simulink model "Ex4_11"  (Simulink 6.0)
settings: Solver=VariableStepDiscrete  StartTime=0.0  StopTime=Tstop  RelTol=1e-3
values from neighbouring files (symbols this model uses):
  Ampl = 10^(Amp_dB/20)*Vfs/2    (= 1)    [Ex4_11_launch.m]
  finrad = Fin*2*pi    (= 11198059.7516)    [Ex4_11_launch.m]
  gain = 1    [Ex4_11_launch.m]
  GAIN1 = 2.0    (= 2)    [Ex4_11_launch.m]
  gain1 = 1    [Ex4_11_launch.m]
  GAIN2 = 2.0    (= 2)    [Ex4_11_launch.m]
  gain2 = 1    [Ex4_11_launch.m]
  GAIN3 = 2.0    (= 2)    [Ex4_11_launch.m]
  gainH = 1    [Ex4_11_launch.m]
  sr = 25000e8    (= 2500000000000)    [Ex4_11_launch.m]
  sr1 = 10000e8    (= 1000000000000)    [Ex4_11_launch.m]
  sr2 = 20000e8    (= 2000000000000)    [Ex4_11_launch.m]
  srH = 250e6    (= 250000000)    [Ex4_11_launch.m]
  tau = 1/(2*pi*beta*f_T)    (= 5.30516476973e-11)    [Ex4_11_launch.m]
  tau1 = 1/(2*pi*beta1*f_T1)    (= 5.30516476973e-11)    [Ex4_11_launch.m]
  tau2 = 1/(2*pi*beta2*f_T2)    (= 5.30516476973e-11)    [Ex4_11_launch.m]
  tauH = 1/(2*pi*betaH*f_TH)    (= 2.65258238486e-10)    [Ex4_11_launch.m]
  Tmax = Ts/2    (= 5e-09)    [Ex4_11_launch.m]
  Ts = 1e-8    (= 1e-08)    [Ex4_11_launch.m]
  V_DAC_H1 = 0.5    [Ex4_11_launch.m]
  V_DAC_H2 = 0.5    [Ex4_11_launch.m]
  V_DAC_H3 = 0.5    [Ex4_11_launch.m]
  V_DAC_L1 = -0.5    [Ex4_11_launch.m]
  V_DAC_L2 = -0.5    [Ex4_11_launch.m]
  V_DAC_L3 = -0.5    [Ex4_11_launch.m]
  VthH1 = 0.25+eps    [Ex4_11_launch.m]
  VthH2 = 0.25+eps    [Ex4_11_launch.m]
  VthH3 = 0.25+eps    [Ex4_11_launch.m]
  VthL1 = -0.25+eps    [Ex4_11_launch.m]
  VthL2 = -0.25+eps    [Ex4_11_launch.m]
  VthL3 = -0.25+eps    [Ex4_11_launch.m]
undefined symbols (not defined in the file or in its folder): RealBuffer
settings Model: Creator=francomaloberti  LastModifiedBy=Cri  ExtModeAutoUpdateStatusClock=off
settings DataIOCC: SignalLoggingName=sigsOut
settings OptimizationCC: InlineInvariantSignals=off
settings DebuggingCC: SolverPrmCheckMsg=none
settings HardwareCC: TargetUnknown=on

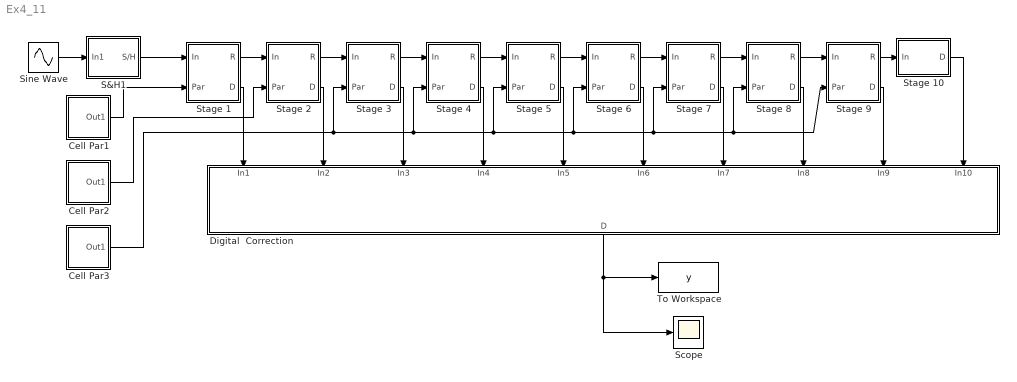
== system Ex4_11 ==
  Cell Par1 : Subsystem
  Cell Par2 : Subsystem
  Cell Par3 : Subsystem
  Digital  Correction : Subsystem  Orientation=down
  S&H1 : Subsystem
  Scope : Scope
  Sine Wave : Sin  Amplitude=Ampl  Frequency=finrad  SampleTime=0
  Stage 1 : Subsystem
  Stage 10 : Subsystem
  Stage 2 : Subsystem
  Stage 3 : Subsystem
  Stage 4 : Subsystem
  Stage 5 : Subsystem
  Stage 6 : Subsystem
  Stage 7 : Subsystem
  Stage 8 : Subsystem
  Stage 9 : Subsystem
  To Workspace : ToWorkspace  VariableName=y  SampleTime=-1  SaveFormat=Array
  wires:
  S&H1/1(S/H) -> Stage 1/1(In)
  Stage 1/1(R) -> Stage 2/1(In)
  Stage 2/1(R) -> Stage 3/1(In)
  Stage 3/1(R) -> Stage 4/1(In)
  Stage 4/1(R) -> Stage 5/1(In)
  Stage 5/1(R) -> Stage 6/1(In)
  Stage 6/1(R) -> Stage 7/1(In)
  Stage 7/1(R) -> Stage 8/1(In)
  Stage 8/1(R) -> Stage 9/1(In)
  Stage 9/1(R) -> Stage 10/1(In)
  Stage 9/2(D) -> Digital  Correction/9(In9)
  Stage 8/2(D) -> Digital  Correction/8(In8)
  Stage 7/2(D) -> Digital  Correction/7(In7)
  Stage 6/2(D) -> Digital  Correction/6(In6)
  Stage 4/2(D) -> Digital  Correction/4(In4)
  Stage 3/2(D) -> Digital  Correction/3(In3)
  Stage 2/2(D) -> Digital  Correction/2(In2)
  Stage 1/2(D) -> Digital  Correction/1(In1)
  Stage 5/2(D) -> Digital  Correction/5(In5)
  Cell Par1/1(Out1) -> Stage 1/2(Par)
  Cell Par2/1(Out1) -> Stage 2/2(Par)
  Cell Par3/1(Out1) -> Stage 3/2(Par), Stage 4/2(Par), Stage 5/2(Par), Stage 6/2(Par), Stage 8/2(Par), Stage 9/2(Par), Stage 7/2(Par)
  Stage 10/1(D) -> Digital  Correction/10(In10)
  Sine Wave/1 -> S&H1/1(In1)
  Digital  Correction/1(D) -> To Workspace/1, Scope/1

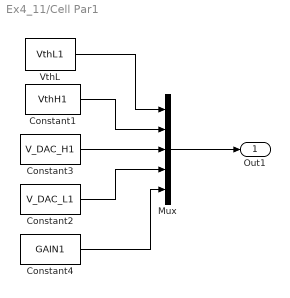
== system Ex4_11/Cell Par1 ==
  Constant1 : Constant  Value=VthH1
  Constant2 : Constant  Value=V_DAC_L1
  Constant3 : Constant  Value=V_DAC_H1
  Constant4 : Constant  Value=GAIN1
  Mux : Mux  Inputs=5
  VthL : Constant  Value=VthL1
  Out1 : Outport
  wires:
  Mux/1 -> Out1/1
  VthL/1 -> Mux/1
  Constant1/1 -> Mux/2
  Constant4/1 -> Mux/5
  Constant3/1 -> Mux/3
  Constant2/1 -> Mux/4

== system Ex4_11/Cell Par2 ==
  Constant1 : Constant  Value=VthH2
  Constant2 : Constant  Value=V_DAC_L2
  Constant3 : Constant  Value=V_DAC_H2
  Constant4 : Constant  Value=GAIN2
  Mux : Mux  Inputs=5
  VthL : Constant  Value=VthL2
  Out1 : Outport
  wires:
  Constant2/1 -> Mux/4
  Constant3/1 -> Mux/3
  Constant4/1 -> Mux/5
  Constant1/1 -> Mux/2
  VthL/1 -> Mux/1
  Mux/1 -> Out1/1

== system Ex4_11/Cell Par3 ==
  Constant1 : Constant  Value=VthH3
  Constant2 : Constant  Value=V_DAC_L3
  Constant3 : Constant  Value=V_DAC_H3
  Constant4 : Constant  Value=GAIN3
  Mux : Mux  Inputs=5
  VthL : Constant  Value=VthL3
  Out1 : Outport
  wires:
  Mux/1 -> Out1/1
  VthL/1 -> Mux/1
  Constant1/1 -> Mux/2
  Constant4/1 -> Mux/5
  Constant3/1 -> Mux/3
  Constant2/1 -> Mux/4

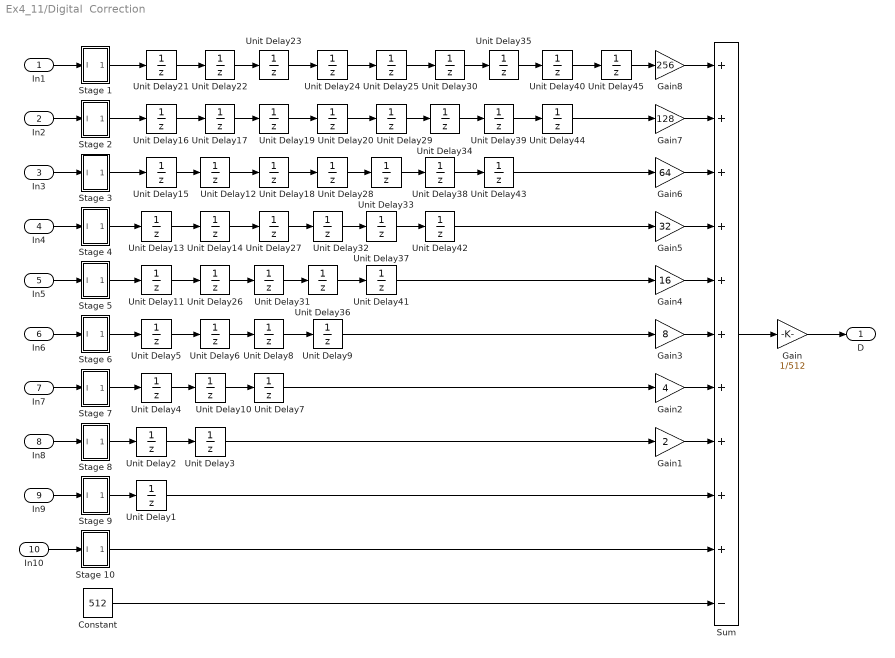
== system Ex4_11/Digital  Correction ==
  In1 : Inport  Port=1  LatchInput=off
  In2 : Inport  Port=2  LatchInput=off
  In3 : Inport  Port=3  LatchInput=off
  In4 : Inport  Port=4  LatchInput=off
  In5 : Inport  Port=5  LatchInput=off
  In6 : Inport  Port=6  LatchInput=off
  In7 : Inport  Port=7  LatchInput=off
  In8 : Inport  Port=8  LatchInput=off
  In9 : Inport  Port=9  LatchInput=off
  In10 : Inport  Port=10  LatchInput=off
  Constant : Constant  Value=512
  Gain : Gain  Gain=1/512
  Gain1 : Gain  Gain=2
  Gain2 : Gain  Gain=4
  Gain3 : Gain  Gain=8
  Gain4 : Gain  Gain=16
  Gain5 : Gain  Gain=32
  Gain6 : Gain  Gain=64
  Gain7 : Gain  Gain=128
  Gain8 : Gain  Gain=256
  Stage 1 : Subsystem
  Stage 10 : Subsystem
  Stage 2 : Subsystem
  Stage 3 : Subsystem
  Stage 4 : Subsystem
  Stage 5 : Subsystem
  Stage 6 : Subsystem
  Stage 7 : Subsystem
  Stage 8 : Subsystem
  Stage 9 : Subsystem
  Sum : Sum  Inputs=++++++++++-
  Unit Delay{1..45} (45 alike) : UnitDelay  SampleTime=Ts
  D : Outport
  wires:
  Gain8/1 -> Sum/1
  Gain7/1 -> Sum/2
  Gain6/1 -> Sum/3
  Gain5/1 -> Sum/4
  Gain4/1 -> Sum/5
  Gain3/1 -> Sum/6
  Gain2/1 -> Sum/7
  Gain1/1 -> Sum/8
  Constant/1 -> Sum/11
  Stage 10/1(D) -> Sum/10
  Unit Delay1/1 -> Sum/9
  Unit Delay3/1 -> Gain1/1
  Unit Delay7/1 -> Gain2/1
  Unit Delay9/1 -> Gain3/1
  Unit Delay41/1 -> Gain4/1
  Unit Delay42/1 -> Gain5/1
  Unit Delay43/1 -> Gain6/1
  Unit Delay44/1 -> Gain7/1
  Unit Delay45/1 -> Gain8/1
  Unit Delay40/1 -> Unit Delay45/1
  Unit Delay35/1 -> Unit Delay40/1
  Unit Delay30/1 -> Unit Delay35/1
  Unit Delay25/1 -> Unit Delay30/1
  Unit Delay39/1 -> Unit Delay44/1
  Unit Delay34/1 -> Unit Delay39/1
  Unit Delay29/1 -> Unit Delay34/1
  Unit Delay20/1 -> Unit Delay29/1
  Unit Delay38/1 -> Unit Delay43/1
  Unit Delay33/1 -> Unit Delay38/1
  Unit Delay28/1 -> Unit Delay33/1
  Unit Delay18/1 -> Unit Delay28/1
  Unit Delay37/1 -> Unit Delay42/1
  Unit Delay32/1 -> Unit Delay37/1
  Unit Delay27/1 -> Unit Delay32/1
  Unit Delay14/1 -> Unit Delay27/1
  Unit Delay36/1 -> Unit Delay41/1
  Unit Delay31/1 -> Unit Delay36/1
  Unit Delay26/1 -> Unit Delay31/1
  Unit Delay11/1 -> Unit Delay26/1
  Unit Delay24/1 -> Unit Delay25/1
  Stage 1/1(D) -> Unit Delay21/1
  Unit Delay22/1 -> Unit Delay23/1
  Unit Delay23/1 -> Unit Delay24/1
  Unit Delay21/1 -> Unit Delay22/1
  Stage 2/1(D) -> Unit Delay16/1
  Stage 3/1(D) -> Unit Delay15/1
  Stage 4/1(D) -> Unit Delay13/1
  Stage 5/1(D) -> Unit Delay11/1
  Unit Delay17/1 -> Unit Delay19/1
  Unit Delay12/1 -> Unit Delay18/1
  Unit Delay15/1 -> Unit Delay12/1
  Unit Delay19/1 -> Unit Delay20/1
  Unit Delay16/1 -> Unit Delay17/1
  Unit Delay13/1 -> Unit Delay14/1
  Unit Delay6/1 -> Unit Delay8/1
  Stage 6/1(D) -> Unit Delay5/1
  Unit Delay10/1 -> Unit Delay7/1
  Unit Delay4/1 -> Unit Delay10/1
  Stage 7/1(D) -> Unit Delay4/1
  Unit Delay8/1 -> Unit Delay9/1
  Unit Delay5/1 -> Unit Delay6/1
  Stage 9/1(D) -> Unit Delay1/1
  Unit Delay2/1 -> Unit Delay3/1
  Stage 8/1(D) -> Unit Delay2/1
  In9/1 -> Stage 9/1(I)
  In8/1 -> Stage 8/1(I)
  In7/1 -> Stage 7/1(I)
  In6/1 -> Stage 6/1(I)
  In5/1 -> Stage 5/1(I)
  In4/1 -> Stage 4/1(I)
  In3/1 -> Stage 3/1(I)
  In2/1 -> Stage 2/1(I)
  In1/1 -> Stage 1/1(I)
  In10/1 -> Stage 10/1(I)
  Gain/1 -> D/1
  Sum/1 -> Gain/1

== system Ex4_11/S&H1 ==
  In1 : Inport  Port=1  LatchInput=off
  Constant : Constant  Value=1/1024-eps
  MATLAB Fcn : MATLABFcn  MATLABFcn=RealBuffer(u,srH,tauH,gainH,Tmax)
  Sum1 : Sum  Inputs=|++  SaturateOnIntegerOverflow=on
  Unit Delay1 : UnitDelay  SampleTime=Ts
  S/H : Outport
  wires:
  Constant/1 -> Sum1/2
  Unit Delay1/1 -> Sum1/1
  Sum1/1 -> MATLAB Fcn/1
  In1/1 -> Unit Delay1/1
  MATLAB Fcn/1 -> S/H/1

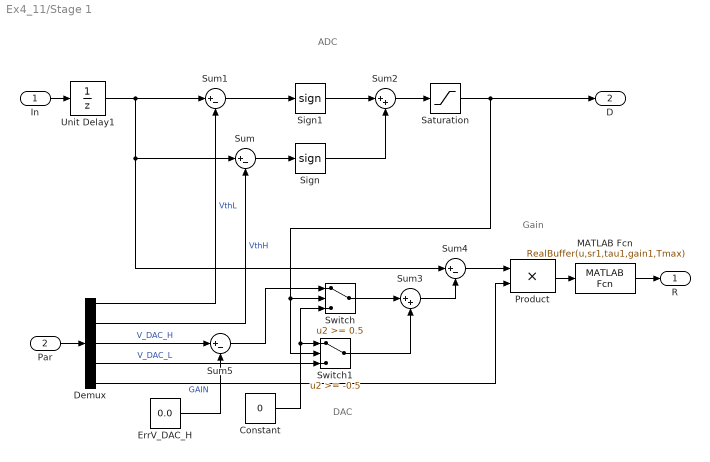
== system Ex4_11/Stage 1 ==
  note: ADC
  note: DAC
  note: Gain
  In : Inport  Port=1  LatchInput=off
  Par : Inport  Port=2  LatchInput=off
  Constant : Constant  Value=0
  Demux : Demux  Outputs=5
  ErrV_DAC_H : Constant  Value=0.0
  MATLAB Fcn : MATLABFcn  MATLABFcn=RealBuffer(u,sr1,tau1,gain1,Tmax)
  Product : Product  SaturateOnIntegerOverflow=on
  Saturation : Saturate  UpperLimit=1  LowerLimit=-1
  Sign : Signum
  Sign1 : Signum
  Sum{,1,4..5} (4 alike) : Sum  Inputs=|+-  SaturateOnIntegerOverflow=on
  Sum2 : Sum  Inputs=|++  SaturateOnIntegerOverflow=on
  Sum3 : Sum  Inputs=|++  SaturateOnIntegerOverflow=on
  Switch : Switch  Threshold=0.5  SaturateOnIntegerOverflow=on
  Switch1 : Switch  Threshold=-0.5  SaturateOnIntegerOverflow=on
  Unit Delay1 : UnitDelay  SampleTime=Ts
  R : Outport
  D : Outport  Port=2
  wires:
  Par/1 -> Demux/1
  Sum/1 -> Sign/1
  Sum1/1 -> Sign1/1
  Demux/1 -> Sum1/2  "VthL"
  Demux/2 -> Sum/2  "VthH"
  In/1 -> Unit Delay1/1
  Sign1/1 -> Sum2/1
  Sign/1 -> Sum2/2
  Sum2/1 -> Saturation/1
  Saturation/1 -> Switch1/2, Switch/2, D/1
  Switch/1 -> Sum3/1
  Switch1/1 -> Sum3/2
  Demux/4 -> Switch1/3  "V_DAC_L"
  Constant/1 -> Switch/3, Switch1/1
  Demux/5 -> Product/2  "GAIN"
  Product/1 -> MATLAB Fcn/1
  Sum3/1 -> Sum4/2
  Sum4/1 -> Product/1
  Demux/3 -> Sum5/1  "V_DAC_H"
  Sum5/1 -> Switch/1
  ErrV_DAC_H/1 -> Sum5/2
  Unit Delay1/1 -> Sum1/1, Sum4/1, Sum/1
  MATLAB Fcn/1 -> R/1

== system Ex4_11/Stage 10 ==
  note: ADC
  In : Inport  Port=1  LatchInput=off
  Sign1 : Signum
  Unit Delay1 : UnitDelay  SampleTime=Ts
  D : Outport
  wires:
  Unit Delay1/1 -> Sign1/1
  Sign1/1 -> D/1
  In/1 -> Unit Delay1/1

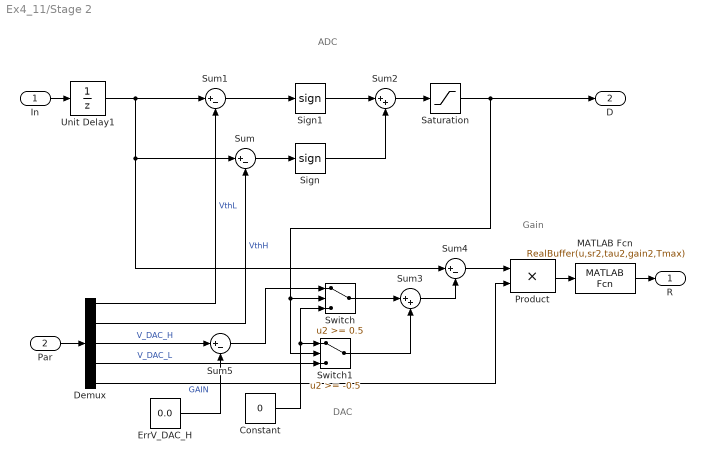
== system Ex4_11/Stage 2 ==
  note: Gain
  note: DAC
  note: ADC
  In : Inport  Port=1  LatchInput=off
  Par : Inport  Port=2  LatchInput=off
  Constant : Constant  Value=0
  Demux : Demux  Outputs=5
  ErrV_DAC_H : Constant  Value=0.0
  MATLAB Fcn : MATLABFcn  MATLABFcn=RealBuffer(u,sr2,tau2,gain2,Tmax)
  Product : Product  SaturateOnIntegerOverflow=on
  Saturation : Saturate  UpperLimit=1  LowerLimit=-1
  Sign : Signum
  Sign1 : Signum
  Sum{,1,4..5} (4 alike) : Sum  Inputs=|+-  SaturateOnIntegerOverflow=on
  Sum2 : Sum  Inputs=|++  SaturateOnIntegerOverflow=on
  Sum3 : Sum  Inputs=|++  SaturateOnIntegerOverflow=on
  Switch : Switch  Threshold=0.5  SaturateOnIntegerOverflow=on
  Switch1 : Switch  Threshold=-0.5  SaturateOnIntegerOverflow=on
  Unit Delay1 : UnitDelay  SampleTime=Ts
  R : Outport
  D : Outport  Port=2
  wires:
  Unit Delay1/1 -> Sum/1, Sum4/1, Sum1/1
  ErrV_DAC_H/1 -> Sum5/2
  Sum5/1 -> Switch/1
  Demux/3 -> Sum5/1  "V_DAC_H"
  Sum4/1 -> Product/1
  Sum3/1 -> Sum4/2
  Product/1 -> MATLAB Fcn/1
  Demux/5 -> Product/2  "GAIN"
  Constant/1 -> Switch1/1, Switch/3
  Demux/4 -> Switch1/3  "V_DAC_L"
  Switch1/1 -> Sum3/2
  Switch/1 -> Sum3/1
  Saturation/1 -> D/1, Switch/2, Switch1/2
  Sum2/1 -> Saturation/1
  Sign/1 -> Sum2/2
  Sign1/1 -> Sum2/1
  In/1 -> Unit Delay1/1
  Demux/2 -> Sum/2  "VthH"
  Demux/1 -> Sum1/2  "VthL"
  Sum1/1 -> Sign1/1
  Sum/1 -> Sign/1
  Par/1 -> Demux/1
  MATLAB Fcn/1 -> R/1

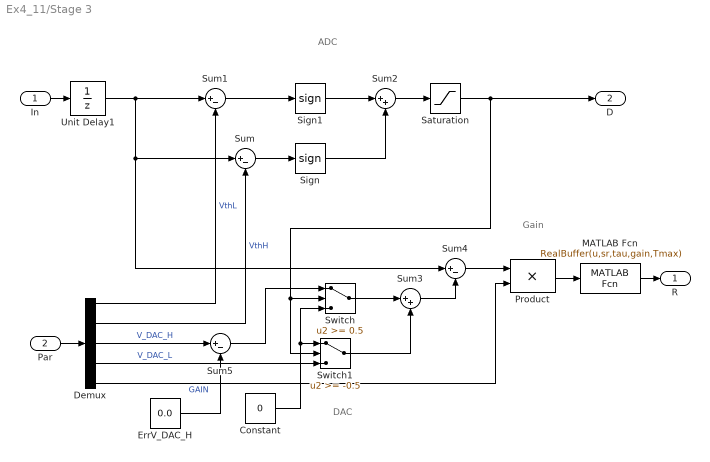
== system Ex4_11/Stage 3 ==
  note: ADC
  note: DAC
  note: Gain
  In : Inport  Port=1  LatchInput=off
  Par : Inport  Port=2  LatchInput=off
  Constant : Constant  Value=0
  Demux : Demux  Outputs=5
  ErrV_DAC_H : Constant  Value=0.0
  MATLAB Fcn : MATLABFcn  MATLABFcn=RealBuffer(u,sr,tau,gain,Tmax)
  Product : Product  SaturateOnIntegerOverflow=on
  Saturation : Saturate  UpperLimit=1  LowerLimit=-1
  Sign : Signum
  Sign1 : Signum
  Sum{,1,4..5} (4 alike) : Sum  Inputs=|+-  SaturateOnIntegerOverflow=on
  Sum2 : Sum  Inputs=|++  SaturateOnIntegerOverflow=on
  Sum3 : Sum  Inputs=|++  SaturateOnIntegerOverflow=on
  Switch : Switch  Threshold=0.5  SaturateOnIntegerOverflow=on
  Switch1 : Switch  Threshold=-0.5  SaturateOnIntegerOverflow=on
  Unit Delay1 : UnitDelay  SampleTime=Ts
  R : Outport
  D : Outport  Port=2
  wires:
  Par/1 -> Demux/1
  Sum/1 -> Sign/1
  Sum1/1 -> Sign1/1
  Demux/1 -> Sum1/2  "VthL"
  Demux/2 -> Sum/2  "VthH"
  In/1 -> Unit Delay1/1
  Sign1/1 -> Sum2/1
  Sign/1 -> Sum2/2
  Sum2/1 -> Saturation/1
  Saturation/1 -> Switch1/2, Switch/2, D/1
  Switch/1 -> Sum3/1
  Switch1/1 -> Sum3/2
  Demux/4 -> Switch1/3  "V_DAC_L"
  Constant/1 -> Switch/3, Switch1/1
  Demux/5 -> Product/2  "GAIN"
  Product/1 -> MATLAB Fcn/1
  Sum3/1 -> Sum4/2
  Sum4/1 -> Product/1
  Demux/3 -> Sum5/1  "V_DAC_H"
  Sum5/1 -> Switch/1
  ErrV_DAC_H/1 -> Sum5/2
  Unit Delay1/1 -> Sum1/1, Sum4/1, Sum/1
  MATLAB Fcn/1 -> R/1

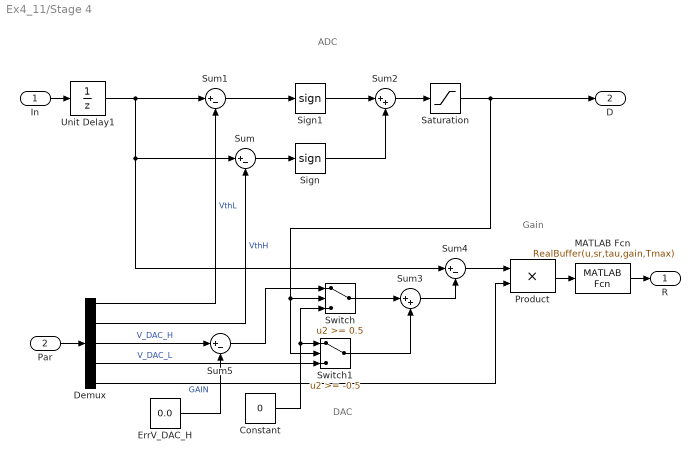
== system Ex4_11/Stage 4 ==
  note: Gain
  note: DAC
  note: ADC
  In : Inport  Port=1  LatchInput=off
  Par : Inport  Port=2  LatchInput=off
  Constant : Constant  Value=0
  Demux : Demux  Outputs=5
  ErrV_DAC_H : Constant  Value=0.0
  MATLAB Fcn : MATLABFcn  MATLABFcn=RealBuffer(u,sr,tau,gain,Tmax)
  Product : Product  SaturateOnIntegerOverflow=on
  Saturation : Saturate  UpperLimit=1  LowerLimit=-1
  Sign : Signum
  Sign1 : Signum
  Sum{,1,4..5} (4 alike) : Sum  Inputs=|+-  SaturateOnIntegerOverflow=on
  Sum2 : Sum  Inputs=|++  SaturateOnIntegerOverflow=on
  Sum3 : Sum  Inputs=|++  SaturateOnIntegerOverflow=on
  Switch : Switch  Threshold=0.5  SaturateOnIntegerOverflow=on
  Switch1 : Switch  Threshold=-0.5  SaturateOnIntegerOverflow=on
  Unit Delay1 : UnitDelay  SampleTime=Ts
  R : Outport
  D : Outport  Port=2
  wires:
  Unit Delay1/1 -> Sum/1, Sum4/1, Sum1/1
  ErrV_DAC_H/1 -> Sum5/2
  Sum5/1 -> Switch/1
  Demux/3 -> Sum5/1  "V_DAC_H"
  Sum4/1 -> Product/1
  Sum3/1 -> Sum4/2
  Product/1 -> MATLAB Fcn/1
  Demux/5 -> Product/2  "GAIN"
  Constant/1 -> Switch1/1, Switch/3
  Demux/4 -> Switch1/3  "V_DAC_L"
  Switch1/1 -> Sum3/2
  Switch/1 -> Sum3/1
  Saturation/1 -> D/1, Switch/2, Switch1/2
  Sum2/1 -> Saturation/1
  Sign/1 -> Sum2/2
  Sign1/1 -> Sum2/1
  In/1 -> Unit Delay1/1
  Demux/2 -> Sum/2  "VthH"
  Demux/1 -> Sum1/2  "VthL"
  Sum1/1 -> Sign1/1
  Sum/1 -> Sign/1
  Par/1 -> Demux/1
  MATLAB Fcn/1 -> R/1

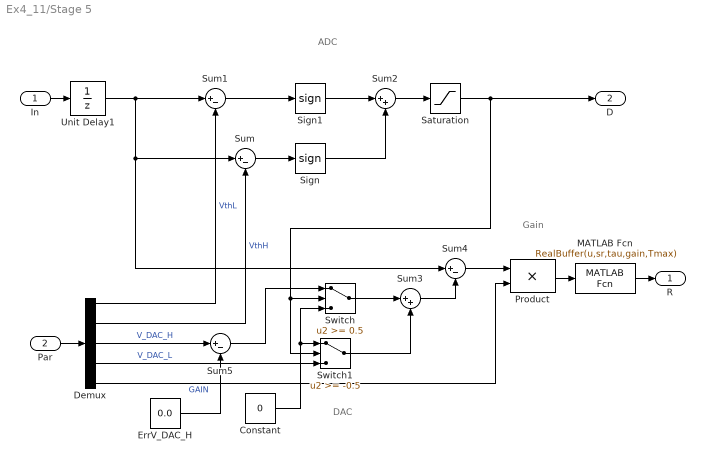
== system Ex4_11/Stage 5 ==
  note: ADC
  note: DAC
  note: Gain
  In : Inport  Port=1  LatchInput=off
  Par : Inport  Port=2  LatchInput=off
  Constant : Constant  Value=0
  Demux : Demux  Outputs=5
  ErrV_DAC_H : Constant  Value=0.0
  MATLAB Fcn : MATLABFcn  MATLABFcn=RealBuffer(u,sr,tau,gain,Tmax)
  Product : Product  SaturateOnIntegerOverflow=on
  Saturation : Saturate  UpperLimit=1  LowerLimit=-1
  Sign : Signum
  Sign1 : Signum
  Sum{,1,4..5} (4 alike) : Sum  Inputs=|+-  SaturateOnIntegerOverflow=on
  Sum2 : Sum  Inputs=|++  SaturateOnIntegerOverflow=on
  Sum3 : Sum  Inputs=|++  SaturateOnIntegerOverflow=on
  Switch : Switch  Threshold=0.5  SaturateOnIntegerOverflow=on
  Switch1 : Switch  Threshold=-0.5  SaturateOnIntegerOverflow=on
  Unit Delay1 : UnitDelay  SampleTime=Ts
  R : Outport
  D : Outport  Port=2
  wires:
  Par/1 -> Demux/1
  Sum/1 -> Sign/1
  Sum1/1 -> Sign1/1
  Demux/1 -> Sum1/2  "VthL"
  Demux/2 -> Sum/2  "VthH"
  In/1 -> Unit Delay1/1
  Sign1/1 -> Sum2/1
  Sign/1 -> Sum2/2
  Sum2/1 -> Saturation/1
  Saturation/1 -> Switch1/2, Switch/2, D/1
  Switch/1 -> Sum3/1
  Switch1/1 -> Sum3/2
  Demux/4 -> Switch1/3  "V_DAC_L"
  Constant/1 -> Switch/3, Switch1/1
  Demux/5 -> Product/2  "GAIN"
  Product/1 -> MATLAB Fcn/1
  Sum3/1 -> Sum4/2
  Sum4/1 -> Product/1
  Demux/3 -> Sum5/1  "V_DAC_H"
  Sum5/1 -> Switch/1
  ErrV_DAC_H/1 -> Sum5/2
  Unit Delay1/1 -> Sum1/1, Sum4/1, Sum/1
  MATLAB Fcn/1 -> R/1

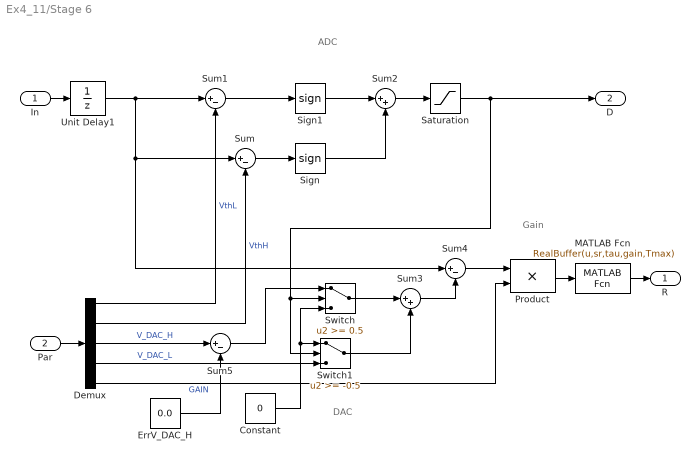
== system Ex4_11/Stage 6 ==
  note: Gain
  note: DAC
  note: ADC
  In : Inport  Port=1  LatchInput=off
  Par : Inport  Port=2  LatchInput=off
  Constant : Constant  Value=0
  Demux : Demux  Outputs=5
  ErrV_DAC_H : Constant  Value=0.0
  MATLAB Fcn : MATLABFcn  MATLABFcn=RealBuffer(u,sr,tau,gain,Tmax)
  Product : Product  SaturateOnIntegerOverflow=on
  Saturation : Saturate  UpperLimit=1  LowerLimit=-1
  Sign : Signum
  Sign1 : Signum
  Sum{,1,4..5} (4 alike) : Sum  Inputs=|+-  SaturateOnIntegerOverflow=on
  Sum2 : Sum  Inputs=|++  SaturateOnIntegerOverflow=on
  Sum3 : Sum  Inputs=|++  SaturateOnIntegerOverflow=on
  Switch : Switch  Threshold=0.5  SaturateOnIntegerOverflow=on
  Switch1 : Switch  Threshold=-0.5  SaturateOnIntegerOverflow=on
  Unit Delay1 : UnitDelay  SampleTime=Ts
  R : Outport
  D : Outport  Port=2
  wires:
  Unit Delay1/1 -> Sum/1, Sum4/1, Sum1/1
  ErrV_DAC_H/1 -> Sum5/2
  Sum5/1 -> Switch/1
  Demux/3 -> Sum5/1  "V_DAC_H"
  Sum4/1 -> Product/1
  Sum3/1 -> Sum4/2
  Product/1 -> MATLAB Fcn/1
  Demux/5 -> Product/2  "GAIN"
  Constant/1 -> Switch1/1, Switch/3
  Demux/4 -> Switch1/3  "V_DAC_L"
  Switch1/1 -> Sum3/2
  Switch/1 -> Sum3/1
  Saturation/1 -> D/1, Switch/2, Switch1/2
  Sum2/1 -> Saturation/1
  Sign/1 -> Sum2/2
  Sign1/1 -> Sum2/1
  In/1 -> Unit Delay1/1
  Demux/2 -> Sum/2  "VthH"
  Demux/1 -> Sum1/2  "VthL"
  Sum1/1 -> Sign1/1
  Sum/1 -> Sign/1
  Par/1 -> Demux/1
  MATLAB Fcn/1 -> R/1

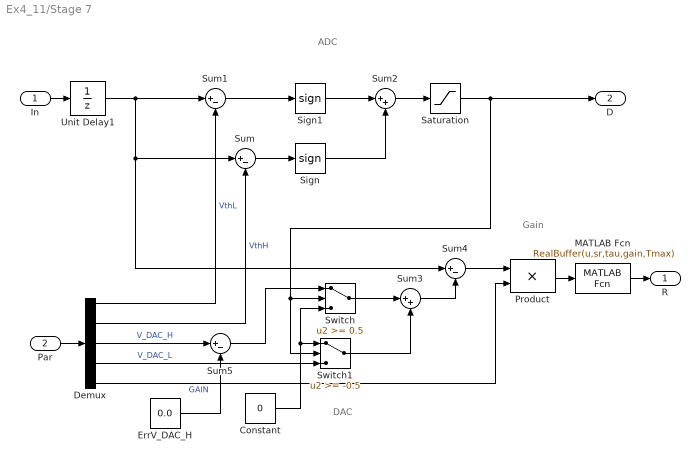
== system Ex4_11/Stage 7 ==
  note: ADC
  note: DAC
  note: Gain
  In : Inport  Port=1  LatchInput=off
  Par : Inport  Port=2  LatchInput=off
  Constant : Constant  Value=0
  Demux : Demux  Outputs=5
  ErrV_DAC_H : Constant  Value=0.0
  MATLAB Fcn : MATLABFcn  MATLABFcn=RealBuffer(u,sr,tau,gain,Tmax)
  Product : Product  SaturateOnIntegerOverflow=on
  Saturation : Saturate  UpperLimit=1  LowerLimit=-1
  Sign : Signum
  Sign1 : Signum
  Sum{,1,4..5} (4 alike) : Sum  Inputs=|+-  SaturateOnIntegerOverflow=on
  Sum2 : Sum  Inputs=|++  SaturateOnIntegerOverflow=on
  Sum3 : Sum  Inputs=|++  SaturateOnIntegerOverflow=on
  Switch : Switch  Threshold=0.5  SaturateOnIntegerOverflow=on
  Switch1 : Switch  Threshold=-0.5  SaturateOnIntegerOverflow=on
  Unit Delay1 : UnitDelay  SampleTime=Ts
  R : Outport
  D : Outport  Port=2
  wires:
  MATLAB Fcn/1 -> R/1
  Par/1 -> Demux/1
  Sum/1 -> Sign/1
  Sum1/1 -> Sign1/1
  Demux/1 -> Sum1/2  "VthL"
  Demux/2 -> Sum/2  "VthH"
  In/1 -> Unit Delay1/1
  Sign1/1 -> Sum2/1
  Sign/1 -> Sum2/2
  Sum2/1 -> Saturation/1
  Saturation/1 -> Switch1/2, Switch/2, D/1
  Switch/1 -> Sum3/1
  Switch1/1 -> Sum3/2
  Demux/4 -> Switch1/3  "V_DAC_L"
  Constant/1 -> Switch/3, Switch1/1
  Demux/5 -> Product/2  "GAIN"
  Product/1 -> MATLAB Fcn/1
  Sum3/1 -> Sum4/2
  Sum4/1 -> Product/1
  Demux/3 -> Sum5/1  "V_DAC_H"
  Sum5/1 -> Switch/1
  ErrV_DAC_H/1 -> Sum5/2
  Unit Delay1/1 -> Sum1/1, Sum4/1, Sum/1

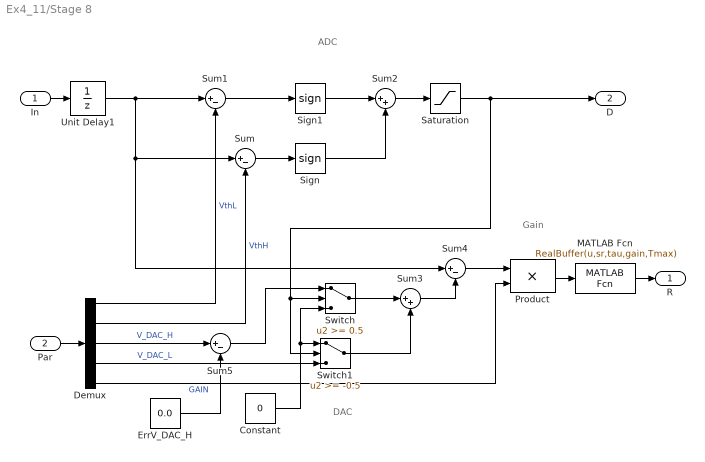
== system Ex4_11/Stage 8 ==
  note: Gain
  note: DAC
  note: ADC
  In : Inport  Port=1  LatchInput=off
  Par : Inport  Port=2  LatchInput=off
  Constant : Constant  Value=0
  Demux : Demux  Outputs=5
  ErrV_DAC_H : Constant  Value=0.0
  MATLAB Fcn : MATLABFcn  MATLABFcn=RealBuffer(u,sr,tau,gain,Tmax)
  Product : Product  SaturateOnIntegerOverflow=on
  Saturation : Saturate  UpperLimit=1  LowerLimit=-1
  Sign : Signum
  Sign1 : Signum
  Sum{,1,4..5} (4 alike) : Sum  Inputs=|+-  SaturateOnIntegerOverflow=on
  Sum2 : Sum  Inputs=|++  SaturateOnIntegerOverflow=on
  Sum3 : Sum  Inputs=|++  SaturateOnIntegerOverflow=on
  Switch : Switch  Threshold=0.5  SaturateOnIntegerOverflow=on
  Switch1 : Switch  Threshold=-0.5  SaturateOnIntegerOverflow=on
  Unit Delay1 : UnitDelay  SampleTime=Ts
  R : Outport
  D : Outport  Port=2
  wires:
  Unit Delay1/1 -> Sum/1, Sum4/1, Sum1/1
  ErrV_DAC_H/1 -> Sum5/2
  Sum5/1 -> Switch/1
  Demux/3 -> Sum5/1  "V_DAC_H"
  Sum4/1 -> Product/1
  Sum3/1 -> Sum4/2
  Product/1 -> MATLAB Fcn/1
  Demux/5 -> Product/2  "GAIN"
  Constant/1 -> Switch1/1, Switch/3
  Demux/4 -> Switch1/3  "V_DAC_L"
  Switch1/1 -> Sum3/2
  Switch/1 -> Sum3/1
  Saturation/1 -> D/1, Switch/2, Switch1/2
  Sum2/1 -> Saturation/1
  Sign/1 -> Sum2/2
  Sign1/1 -> Sum2/1
  In/1 -> Unit Delay1/1
  Demux/2 -> Sum/2  "VthH"
  Demux/1 -> Sum1/2  "VthL"
  Sum1/1 -> Sign1/1
  Sum/1 -> Sign/1
  Par/1 -> Demux/1
  MATLAB Fcn/1 -> R/1

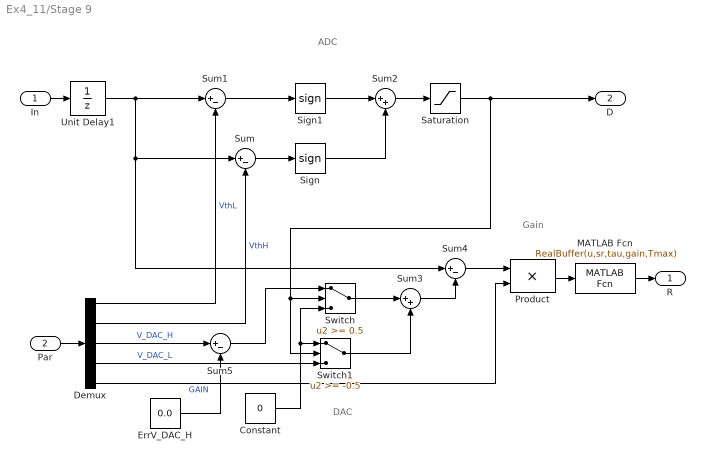
== system Ex4_11/Stage 9 ==
  note: ADC
  note: DAC
  note: Gain
  In : Inport  Port=1  LatchInput=off
  Par : Inport  Port=2  LatchInput=off
  Constant : Constant  Value=0
  Demux : Demux  Outputs=5
  ErrV_DAC_H : Constant  Value=0.0
  MATLAB Fcn : MATLABFcn  MATLABFcn=RealBuffer(u,sr,tau,gain,Tmax)
  Product : Product  SaturateOnIntegerOverflow=on
  Saturation : Saturate  UpperLimit=1  LowerLimit=-1
  Sign : Signum
  Sign1 : Signum
  Sum{,1,4..5} (4 alike) : Sum  Inputs=|+-  SaturateOnIntegerOverflow=on
  Sum2 : Sum  Inputs=|++  SaturateOnIntegerOverflow=on
  Sum3 : Sum  Inputs=|++  SaturateOnIntegerOverflow=on
  Switch : Switch  Threshold=0.5  SaturateOnIntegerOverflow=on
  Switch1 : Switch  Threshold=-0.5  SaturateOnIntegerOverflow=on
  Unit Delay1 : UnitDelay  SampleTime=Ts
  R : Outport
  D : Outport  Port=2
  wires:
  Par/1 -> Demux/1
  Sum/1 -> Sign/1
  Sum1/1 -> Sign1/1
  Demux/1 -> Sum1/2  "VthL"
  Demux/2 -> Sum/2  "VthH"
  In/1 -> Unit Delay1/1
  Sign1/1 -> Sum2/1
  Sign/1 -> Sum2/2
  Sum2/1 -> Saturation/1
  Saturation/1 -> Switch1/2, Switch/2, D/1
  Switch/1 -> Sum3/1
  Switch1/1 -> Sum3/2
  Demux/4 -> Switch1/3  "V_DAC_L"
  Constant/1 -> Switch/3, Switch1/1
  Demux/5 -> Product/2  "GAIN"
  Product/1 -> MATLAB Fcn/1
  Sum3/1 -> Sum4/2
  Sum4/1 -> Product/1
  Demux/3 -> Sum5/1  "V_DAC_H"
  Sum5/1 -> Switch/1
  ErrV_DAC_H/1 -> Sum5/2
  Unit Delay1/1 -> Sum1/1, Sum4/1, Sum/1
  MATLAB Fcn/1 -> R/1

== system Ex4_11/Digital  Correction/Stage 1 ==
  I : Inport  Port=1  LatchInput=off
  Constant : Constant
  Gain : Gain
  Sum : Sum  Inputs=|++
  D : Outport
  wires:
  Gain/1 -> D/1
  I/1 -> Sum/1
  Constant/1 -> Sum/2
  Sum/1 -> Gain/1

== system Ex4_11/Digital  Correction/Stage 10 ==
  I : Inport  Port=1  LatchInput=off
  Constant : Constant
  Gain : Gain  Gain=1/2
  Sum : Sum  Inputs=|++
  D : Outport
  wires:
  Sum/1 -> Gain/1
  Constant/1 -> Sum/2
  I/1 -> Sum/1
  Gain/1 -> D/1

== system Ex4_11/Digital  Correction/Stage 2 ==
  I : Inport  Port=1  LatchInput=off
  Constant : Constant
  Gain : Gain
  Sum : Sum  Inputs=|++
  D : Outport
  wires:
  Sum/1 -> Gain/1
  Constant/1 -> Sum/2
  I/1 -> Sum/1
  Gain/1 -> D/1

== system Ex4_11/Digital  Correction/Stage 3 ==
  I : Inport  Port=1  LatchInput=off
  Constant : Constant
  Gain : Gain
  Sum : Sum  Inputs=|++
  D : Outport
  wires:
  Gain/1 -> D/1
  I/1 -> Sum/1
  Constant/1 -> Sum/2
  Sum/1 -> Gain/1

== system Ex4_11/Digital  Correction/Stage 4 ==
  I : Inport  Port=1  LatchInput=off
  Constant : Constant
  Gain : Gain
  Sum : Sum  Inputs=|++
  D : Outport
  wires:
  Sum/1 -> Gain/1
  Constant/1 -> Sum/2
  I/1 -> Sum/1
  Gain/1 -> D/1

== system Ex4_11/Digital  Correction/Stage 5 ==
  I : Inport  Port=1  LatchInput=off
  Constant : Constant
  Gain : Gain
  Sum : Sum  Inputs=|++
  D : Outport
  wires:
  Gain/1 -> D/1
  I/1 -> Sum/1
  Constant/1 -> Sum/2
  Sum/1 -> Gain/1

== system Ex4_11/Digital  Correction/Stage 6 ==
  I : Inport  Port=1  LatchInput=off
  Constant : Constant
  Gain : Gain
  Sum : Sum  Inputs=|++
  D : Outport
  wires:
  Sum/1 -> Gain/1
  Constant/1 -> Sum/2
  I/1 -> Sum/1
  Gain/1 -> D/1

== system Ex4_11/Digital  Correction/Stage 7 ==
  I : Inport  Port=1  LatchInput=off
  Constant : Constant
  Gain : Gain
  Sum : Sum  Inputs=|++
  D : Outport
  wires:
  Gain/1 -> D/1
  I/1 -> Sum/1
  Constant/1 -> Sum/2
  Sum/1 -> Gain/1

== system Ex4_11/Digital  Correction/Stage 8 ==
  I : Inport  Port=1  LatchInput=off
  Constant : Constant
  Gain : Gain
  Sum : Sum  Inputs=|++
  D : Outport
  wires:
  Sum/1 -> Gain/1
  Constant/1 -> Sum/2
  I/1 -> Sum/1
  Gain/1 -> D/1

== system Ex4_11/Digital  Correction/Stage 9 ==
  I : Inport  Port=1  LatchInput=off
  Constant : Constant
  Gain : Gain
  Sum : Sum  Inputs=|++
  D : Outport
  wires:
  Gain/1 -> D/1
  I/1 -> Sum/1
  Constant/1 -> Sum/2
  Sum/1 -> Gain/1
